simulink model "Appl_MassageMode_CtrlModel"  (R2018b)
settings: configuration reference "CodeConfig_10_ms" (kept outside this file)
undefined symbols (not defined in the file): D_ActMax, D_T1, D_T2, D_T3, D_T4, enMassageLevel_DSM, FALSE, TRUE
libraries: DareLib x33, simulink x1
settings Model: Creator=Administrator  LastModifiedBy=Administrator
settings ConfigSetRef: SourceLocation=Base Workspace

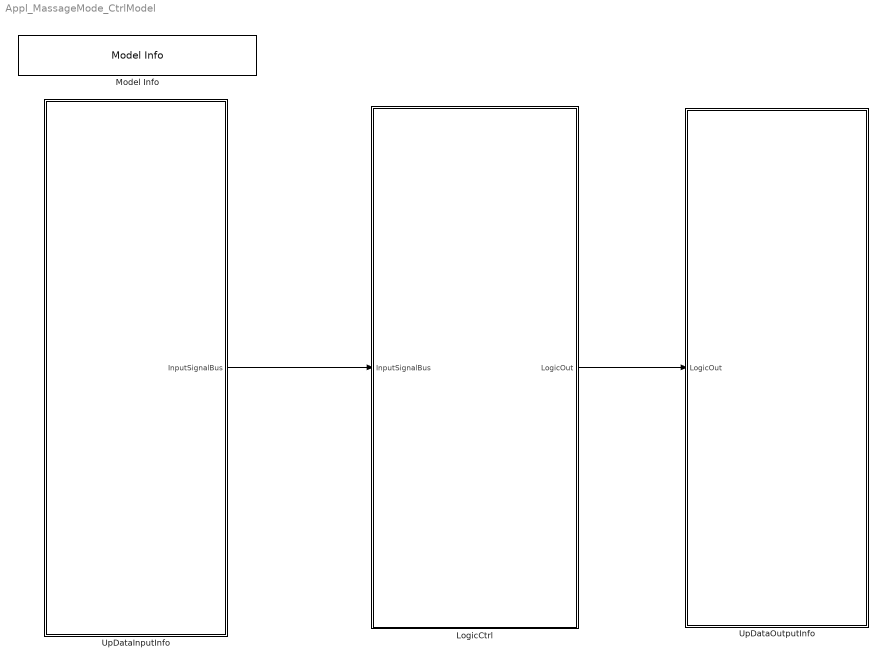
== system Appl_MassageMode_CtrlModel ==
  LogicCtrl : Subsystem  Priority=2  TreatAsAtomicUnit=on
      settings: RTWSystemCode=Nonreusable function  RTWFcnNameOpts=Use subsystem name
  Model Info : simulink/Model-Wide Utilities/Model Info  Frame=on  DisplayStringWithTags=Version：%<ModelVersion>  HorizontalTextAlignment=Center  LeftAlignmentValue=0.5
  UpDataInputInfo : Subsystem  Priority=1  TreatAsAtomicUnit=on
      settings: RTWSystemCode=Nonreusable function  RTWFcnNameOpts=Use subsystem name
  UpDataOutputInfo : Subsystem  Priority=3  TreatAsAtomicUnit=on
      settings: RTWSystemCode=Nonreusable function  RTWFcnNameOpts=Use subsystem name
  wires:
  LogicCtrl/1(LogicOut) -> UpDataOutputInfo/1(LogicOut)
  UpDataInputInfo/1(InputSignalBus) -> LogicCtrl/1(InputSignalBus)

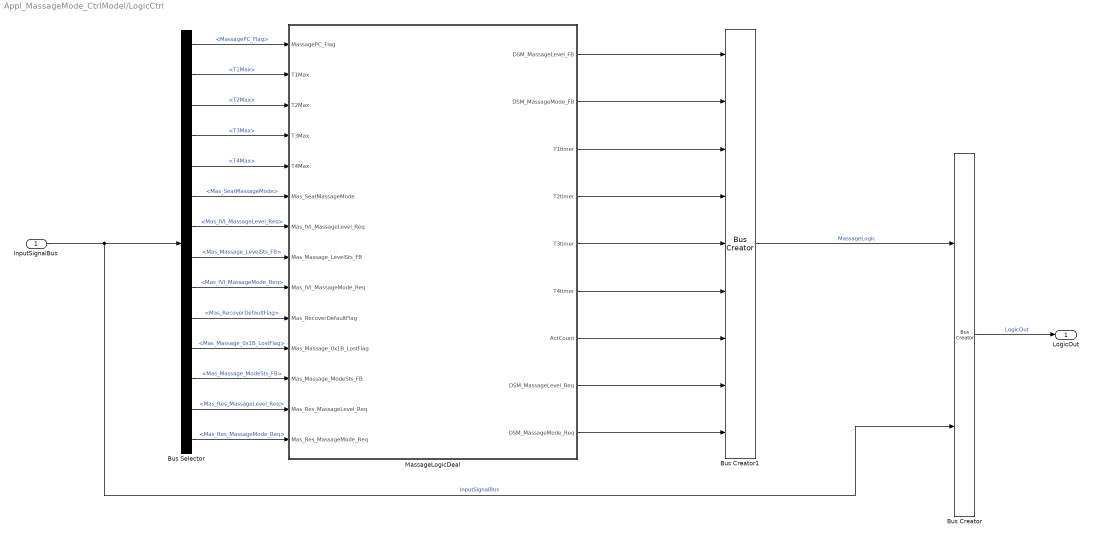
== system Appl_MassageMode_CtrlModel/LogicCtrl ==
  InputSignalBus : Inport
  Bus Creator : BusCreator  Inputs=2
  Bus Creator1 : BusCreator  Inputs=9
  Bus Selector : BusSelector  OutputSignals=MassagePrecondition.MassagePC_Flag,Threshold.T1Max,Threshold.T2Max,Threshold.T3Max,Threshold.T4Max,Rte_SignalBus1.Mas_SeatMassageMode,Rte_SignalBus1.Mas_IVI_MassageLevel_Req,Mas_Massage_LevelSts_FB,Rte_SignalBus1.Mas_IVI_MassageMode_Req,Rte_SignalBus1.Mas_RecoverDefaultFlag,Rte_SignalBus1.Mas_Massage_0x1B_LostFlag,Rte_SignalBus1.Mas_Massage_ModeSts_FB,Rte_SignalBus1.Mas_Res_MassageLevel_Req,Rte_SignalBus1.Mas_Res_MassageMode_Req
  MassageLogicDeal : Subsystem  Description=按摩逻辑处理
      settings: AttributesFormatString=%<Description>
  LogicOut : Outport
  wires:
  InputSignalBus/1 -> Bus Creator/2, Bus Selector/1  "InputSignalBus"
  Bus Creator/1 -> LogicOut/1  "LogicOut"
  MassageLogicDeal/7(ActCount) -> Bus Creator1/7
  MassageLogicDeal/6(T4timer) -> Bus Creator1/6
  MassageLogicDeal/8(DSM_MassageLevel_Req) -> Bus Creator1/8
  MassageLogicDeal/5(T3timer) -> Bus Creator1/5
  MassageLogicDeal/9(DSM_MassageMode_Req) -> Bus Creator1/9
  MassageLogicDeal/4(T2timer) -> Bus Creator1/4
  MassageLogicDeal/3(T1timer) -> Bus Creator1/3
  MassageLogicDeal/2(DSM_MassageMode_FB) -> Bus Creator1/2
  MassageLogicDeal/1(DSM_MassageLevel_FB) -> Bus Creator1/1
  Bus Creator1/1 -> Bus Creator/1  "MassageLogic"
  Bus Selector/1 -> MassageLogicDeal/1(MassagePC_Flag)  "<MassagePC_Flag>"
  Bus Selector/2 -> MassageLogicDeal/2(T1Max)  "<T1Max>"
  Bus Selector/3 -> MassageLogicDeal/3(T2Max)  "<T2Max>"
  Bus Selector/4 -> MassageLogicDeal/4(T3Max)  "<T3Max>"
  Bus Selector/5 -> MassageLogicDeal/5(T4Max)  "<T4Max>"
  Bus Selector/6 -> MassageLogicDeal/6(Mas_SeatMassageMode)  "<Mas_SeatMassageMode>"
  Bus Selector/7 -> MassageLogicDeal/7(Mas_IVI_MassageLevel_Req)  "<Mas_IVI_MassageLevel_Req>"
  Bus Selector/8 -> MassageLogicDeal/8(Mas_Massage_LevelSts_FB)  "<Mas_Massage_LevelSts_FB>"
  Bus Selector/9 -> MassageLogicDeal/9(Mas_IVI_MassageMode_Req)  "<Mas_IVI_MassageMode_Req>"
  Bus Selector/10 -> MassageLogicDeal/10(Mas_RecoverDefaultFlag)  "<Mas_RecoverDefaultFlag>"
  Bus Selector/11 -> MassageLogicDeal/11(Mas_Massage_0x1B_LostFlag)  "<Mas_Massage_0x1B_LostFlag>"
  Bus Selector/12 -> MassageLogicDeal/12(Mas_Massage_ModeSts_FB)  "<Mas_Massage_ModeSts_FB>"
  Bus Selector/13 -> MassageLogicDeal/13(Mas_Res_MassageLevel_Req)  "<Mas_Res_MassageLevel_Req>"
  Bus Selector/14 -> MassageLogicDeal/14(Mas_Res_MassageMode_Req)  "<Mas_Res_MassageMode_Req>"

== system Appl_MassageMode_CtrlModel/UpDataInputInfo ==
  InputSignalProcess : Subsystem  Description=预处理
      settings: AttributesFormatString=%<Description>  RTWSystemCode=Nonreusable function  RTWFcnNameOpts=Use subsystem name
  RTE : Subsystem  Description=接口自动生成  TreatAsAtomicUnit=on
      settings: AttributesFormatString=%<Description>  RTWSystemCode=Nonreusable function  RTWFcnNameOpts=Use subsystem name
  InputSignalBus : Outport
  wires:
  RTE/1(RTE_Signal) -> InputSignalProcess/1(Rte_SignalBus)
  InputSignalProcess/1(InputSignalBus) -> InputSignalBus/1

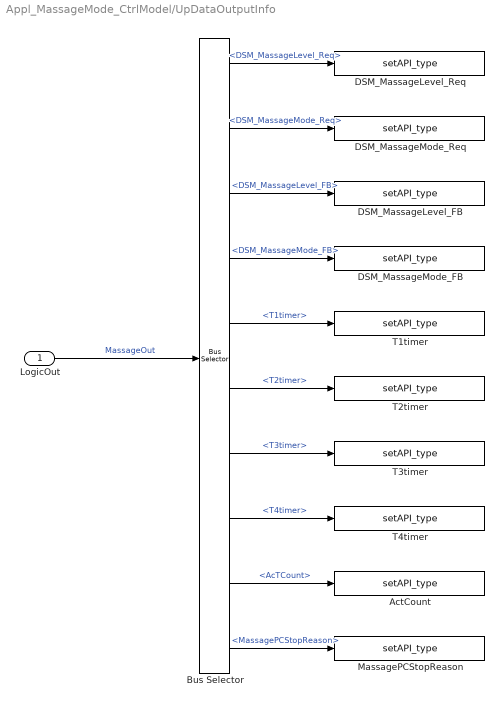
== system Appl_MassageMode_CtrlModel/UpDataOutputInfo ==
  LogicOut : Inport
  ActCount : DareLib/Dare/setAPI_type  g_funcname=Rte_SetVfb_Debug_Mas_ActCount  g_param=""  g_type=uint8  g_size=-1
      settings: AttributesFormatString=%<g_funcname>  SourceProductName=Dare Library
  Bus Selector : BusSelector  OutputSignals=MassageLogic.DSM_MassageLevel_Req,MassageLogic.DSM_MassageMode_Req,MassageLogic.DSM_MassageLevel_FB,MassageLogic.DSM_MassageMode_FB,MassageLogic.T1timer,MassageLogic.T2timer,MassageLogic.T3timer,MassageLogic.T4timer,MassageLogic.AcTCount,InputSignalBus.MassagePrecondition.MassagePCStopReason
  DSM_MassageLevel_FB : DareLib/Dare/setAPI_type  g_funcname=CanTx_0x3B2_DSM_MassageLevel_FB  g_param=""  g_type=uint8  g_enum=enMassageLevel_DSM  g_size=-1
      settings: AttributesFormatString=%<g_funcname>  SourceProductName=Dare Library
  DSM_MassageLevel_Req : DareLib/Dare/setAPI_type  g_funcname=LinSignalSet_DSM_1_1_DSM_MassageLevel_Req  g_param=""  g_type=uint8  g_enum=enMassageLevel_DSM  g_size=-1
      settings: AttributesFormatString=%<g_funcname>  SourceProductName=Dare Library
  DSM_MassageMode_FB : DareLib/Dare/setAPI_type  g_funcname=CanTx_0x3B2_DSM_MassageMode_FB  g_param=""  g_type=uint8  g_enum=enMassageMode_DSM  g_size=-1
      settings: AttributesFormatString=%<g_funcname>  SourceProductName=Dare Library
  DSM_MassageMode_Req : DareLib/Dare/setAPI_type  g_funcname=LinSignalSet_DSM_1_1_DSM_MassageMode_Req  g_param=""  g_type=uint8  g_enum=enMassageMode_DSM  g_size=-1
      settings: AttributesFormatString=%<g_funcname>  SourceProductName=Dare Library
  MassagePCStopReason : DareLib/Dare/setAPI_type  g_funcname=Rte_SetVfb_Debug_Mas_MassagePCStopReason  g_param=""  g_type=uint8  g_size=-1
      settings: AttributesFormatString=%<g_funcname>  SourceProductName=Dare Library
  T1timer : DareLib/Dare/setAPI_type  g_funcname=Rte_SetVfb_Debug_Mas_T1timer  g_param=""  g_type=uint16  g_size=-1
      settings: AttributesFormatString=%<g_funcname>  SourceProductName=Dare Library
  T2timer : DareLib/Dare/setAPI_type  g_funcname=Rte_SetVfb_Debug_Mas_T2timer  g_param=""  g_type=uint16  g_size=-1
      settings: AttributesFormatString=%<g_funcname>  SourceProductName=Dare Library
  T3timer : DareLib/Dare/setAPI_type  g_funcname=Rte_SetVfb_Debug_Mas_T3timer  g_param=""  g_type=uint32  g_size=-1
      settings: AttributesFormatString=%<g_funcname>  SourceProductName=Dare Library
  T4timer : DareLib/Dare/setAPI_type  g_funcname=Rte_SetVfb_Debug_Mas_T4timer  g_param=""  g_type=uint32  g_size=-1
      settings: AttributesFormatString=%<g_funcname>  SourceProductName=Dare Library
  wires:
  LogicOut/1 -> Bus Selector/1  "MassageOut"
  Bus Selector/4 -> DSM_MassageMode_FB/1  "<DSM_MassageMode_FB>"
  Bus Selector/3 -> DSM_MassageLevel_FB/1  "<DSM_MassageLevel_FB>"
  Bus Selector/5 -> T1timer/1  "<T1timer>"
  Bus Selector/2 -> DSM_MassageMode_Req/1  "<DSM_MassageMode_Req>"
  Bus Selector/6 -> T2timer/1  "<T2timer>"
  Bus Selector/1 -> DSM_MassageLevel_Req/1  "<DSM_MassageLevel_Req>"
  Bus Selector/7 -> T3timer/1  "<T3timer>"
  Bus Selector/8 -> T4timer/1  "<T4timer>"
  Bus Selector/9 -> ActCount/1  "<AcTCount>"
  Bus Selector/10 -> MassagePCStopReason/1  "<MassagePCStopReason>"

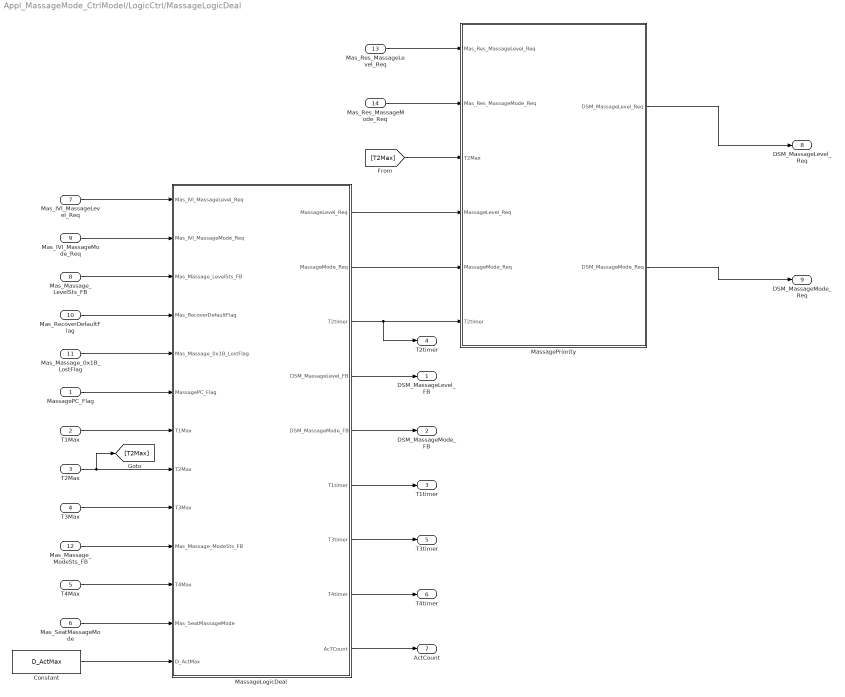
== system Appl_MassageMode_CtrlModel/LogicCtrl/MassageLogicDeal ==
  MassagePC_Flag : Inport
  T1Max : Inport  Port=2
  T2Max : Inport  Port=3
  T3Max : Inport  Port=4
  T4Max : Inport  Port=5
  Mas_SeatMassageMode : Inport  Port=6
  Mas_IVI_MassageLevel_Req : Inport  Port=7
  Mas_Massage_LevelSts_FB : Inport  Port=8
  Mas_IVI_MassageMode_Req : Inport  Port=9
  Mas_RecoverDefaultFlag : Inport  Port=10
  Mas_Massage_0x1B_LostFlag : Inport  Port=11
  Mas_Massage_ModeSts_FB : Inport  Port=12
  Mas_Res_MassageLevel_Req : Inport  Port=13
  Mas_Res_MassageMode_Req : Inport  Port=14
  Constant : Constant  Value=D_ActMax
  MassageLogicDeal : Stateflow chart  TreatAsAtomicUnit=on
  MassagePriority : Stateflow chart  TreatAsAtomicUnit=on
  DSM_MassageLevel_FB : Outport
  DSM_MassageMode_FB : Outport  Port=2
  T1timer : Outport  Port=3
  T2timer : Outport  Port=4
  T3timer : Outport  Port=5
  T4timer : Outport  Port=6
  ActCount : Outport  Port=7
  DSM_MassageLevel_Req : Outport  Port=8
  DSM_MassageMode_Req : Outport  Port=9
  wires:
  MassagePC_Flag/1 -> MassageLogicDeal/6(MassagePC_Flag)
  T1Max/1 -> MassageLogicDeal/7(T1Max)
  T2Max/1 -> [T2Max], MassageLogicDeal/8(T2Max)
  T3Max/1 -> MassageLogicDeal/9(T3Max)
  T4Max/1 -> MassageLogicDeal/11(T4Max)
  MassageLogicDeal/1(MassageLevel_Req) -> MassagePriority/4(MassageLevel_Req)
  MassageLogicDeal/2(MassageMode_Req) -> MassagePriority/5(MassageMode_Req)
  MassageLogicDeal/4(DSM_MassageLevel_FB) -> DSM_MassageLevel_FB/1
  Mas_IVI_MassageMode_Req/1 -> MassageLogicDeal/2(Mas_IVI_MassageMode_Req)
  Mas_RecoverDefaultFlag/1 -> MassageLogicDeal/4(Mas_RecoverDefaultFlag)
  Mas_Massage_0x1B_LostFlag/1 -> MassageLogicDeal/5(Mas_Massage_0x1B_LostFlag)
  Mas_Massage_ModeSts_FB/1 -> MassageLogicDeal/10(Mas_Massage_ModeSts_FB)
  Mas_Massage_LevelSts_FB/1 -> MassageLogicDeal/3(Mas_Massage_LevelSts_FB)
  Mas_IVI_MassageLevel_Req/1 -> MassageLogicDeal/1(Mas_IVI_MassageLevel_Req)
  MassageLogicDeal/7(T3timer) -> T3timer/1
  MassageLogicDeal/3(T2timer) -> T2timer/1, MassagePriority/6(T2timer)
  MassageLogicDeal/6(T1timer) -> T1timer/1
  MassageLogicDeal/5(DSM_MassageMode_FB) -> DSM_MassageMode_FB/1
  Mas_SeatMassageMode/1 -> MassageLogicDeal/12(Mas_SeatMassageMode)
  MassageLogicDeal/8(T4timer) -> T4timer/1
  MassageLogicDeal/9(AcTCount) -> ActCount/1
  Constant/1 -> MassageLogicDeal/13(D_ActMax)
  MassagePriority/2(DSM_MassageMode_Req) -> DSM_MassageMode_Req/1
  MassagePriority/1(DSM_MassageLevel_Req) -> DSM_MassageLevel_Req/1
  Mas_Res_MassageLevel_Req/1 -> MassagePriority/1(Mas_Res_MassageLevel_Req)
  Mas_Res_MassageMode_Req/1 -> MassagePriority/2(Mas_Res_MassageMode_Req)
  [T2Max] -> MassagePriority/3(T2Max)

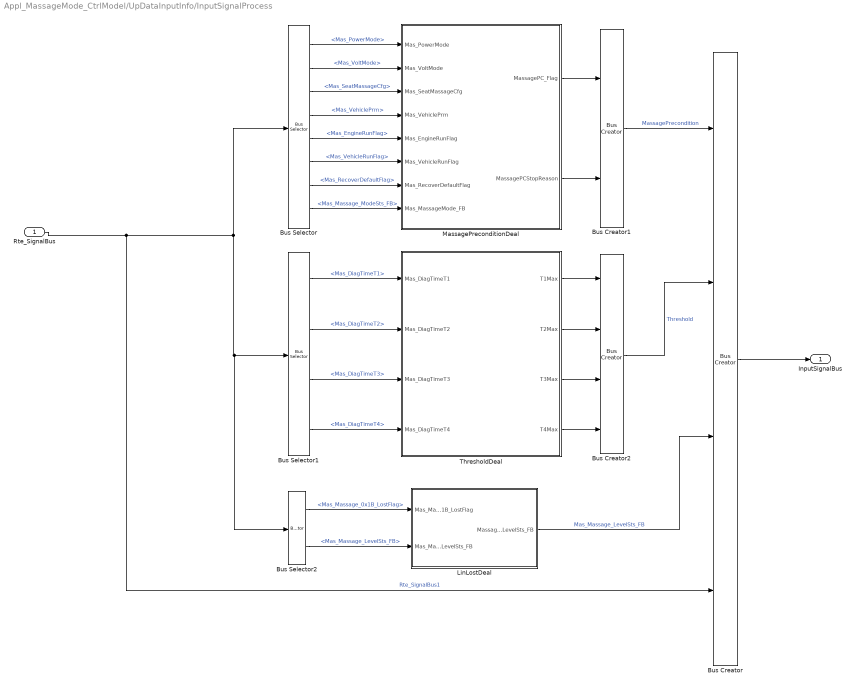
== system Appl_MassageMode_CtrlModel/UpDataInputInfo/InputSignalProcess ==
  Rte_SignalBus : Inport
  Bus Creator : BusCreator  Inputs=4
  Bus Creator1 : BusCreator  Inputs=2
  Bus Creator2 : BusCreator  Inputs=4
  Bus Selector : BusSelector  OutputSignals=Mas_PowerMode,Mas_VoltMode,Mas_SeatMassageCfg,Mas_VehiclePrm,Mas_EngineRunFlag,Mas_VehicleRunFlag,Mas_RecoverDefaultFlag,Mas_Massage_ModeSts_FB
  Bus Selector1 : BusSelector  OutputSignals=Mas_DiagTimeT1,Mas_DiagTimeT2,Mas_DiagTimeT3,Mas_DiagTimeT4
  Bus Selector2 : BusSelector  OutputSignals=Mas_Massage_0x1B_LostFlag,Mas_Massage_LevelSts_FB
  LinLostDeal : Subsystem  Description=LIN节点掉线处理
      settings: AttributesFormatString=%<Description>
  MassagePreconditionDeal : Subsystem  Description=按摩前置条件处理
      settings: AttributesFormatString=%<Description>
  ThresholdDeal : Subsystem  Description=时间阈值配置处理
      settings: AttributesFormatString=%<Description>
  InputSignalBus : Outport
  wires:
  Bus Creator/1 -> InputSignalBus/1
  Rte_SignalBus/1 -> Bus Creator/4, Bus Selector/1, Bus Selector2/1, Bus Selector1/1  "Rte_SignalBus1"
  MassagePreconditionDeal/1(MassagePC_Flag) -> Bus Creator1/1
  MassagePreconditionDeal/2(MassagePCStopReason) -> Bus Creator1/2
  Bus Selector1/1 -> ThresholdDeal/1(Mas_DiagTimeT1)  "<Mas_DiagTimeT1>"
  Bus Selector1/2 -> ThresholdDeal/2(Mas_DiagTimeT2)  "<Mas_DiagTimeT2>"
  Bus Selector1/3 -> ThresholdDeal/3(Mas_DiagTimeT3)  "<Mas_DiagTimeT3>"
  Bus Selector1/4 -> ThresholdDeal/4(Mas_DiagTimeT4)  "<Mas_DiagTimeT4>"
  ThresholdDeal/1(T1Max) -> Bus Creator2/1
  ThresholdDeal/2(T2Max) -> Bus Creator2/2
  ThresholdDeal/3(T3Max) -> Bus Creator2/3
  ThresholdDeal/4(T4Max) -> Bus Creator2/4
  Bus Selector/1 -> MassagePreconditionDeal/1(Mas_PowerMode)  "<Mas_PowerMode>"
  Bus Selector/2 -> MassagePreconditionDeal/2(Mas_VoltMode)  "<Mas_VoltMode>"
  Bus Selector/3 -> MassagePreconditionDeal/3(Mas_SeatMassageCfg)  "<Mas_SeatMassageCfg>"
  Bus Selector/4 -> MassagePreconditionDeal/4(Mas_VehiclePrm)  "<Mas_VehiclePrm>"
  Bus Selector/5 -> MassagePreconditionDeal/5(Mas_EngineRunFlag)  "<Mas_EngineRunFlag>"
  Bus Selector/6 -> MassagePreconditionDeal/6(Mas_VehicleRunFlag)  "<Mas_VehicleRunFlag>"
  Bus Selector/7 -> MassagePreconditionDeal/7(Mas_RecoverDefaultFlag)  "<Mas_RecoverDefaultFlag>"
  Bus Selector/8 -> MassagePreconditionDeal/8(Mas_MassageMode_FB)  "<Mas_Massage_ModeSts_FB>"
  Bus Creator1/1 -> Bus Creator/1  "MassagePrecondition"
  Bus Creator2/1 -> Bus Creator/2  "Threshold"
  Bus Selector2/1 -> LinLostDeal/1(Mas_Massage_0x1B_LostFlag)  "<Mas_Massage_0x1B_LostFlag>"
  Bus Selector2/2 -> LinLostDeal/2(Mas_Massage_LevelSts_FB)  "<Mas_Massage_LevelSts_FB>"
  LinLostDeal/1(Massage_LevelSts_FB) -> Bus Creator/3  "Mas_Massage_LevelSts_FB"

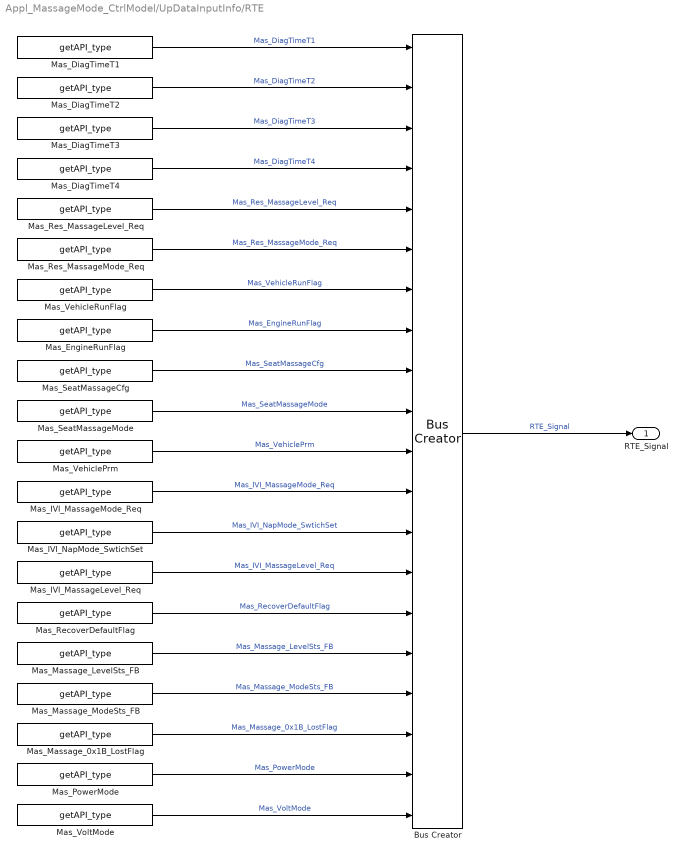
== system Appl_MassageMode_CtrlModel/UpDataInputInfo/RTE ==
  Bus Creator : BusCreator  Inputs=20
  Mas_DiagTimeT1 : DareLib/Dare/getAPI_type  g_funcname=Rte_GetVfb_Debug_Mas_T1_Threshold  g_param=""  g_type=uint16  g_size=-1
      settings: AttributesFormatString=%<g_funcname>  SourceProductName=Dare Library
  Mas_DiagTimeT2 : DareLib/Dare/getAPI_type  g_funcname=Rte_GetVfb_Debug_Mas_T2_Threshold  g_param=""  g_type=uint16  g_size=-1
      settings: AttributesFormatString=%<g_funcname>  SourceProductName=Dare Library
  Mas_DiagTimeT3 : DareLib/Dare/getAPI_type  g_funcname=Rte_GetVfb_Debug_Mas_T3_Threshold  g_param=""  g_type=uint16  g_size=-1
      settings: AttributesFormatString=%<g_funcname>  SourceProductName=Dare Library
  Mas_DiagTimeT4 : DareLib/Dare/getAPI_type  g_funcname=Rte_GetVfb_Debug_Mas_T4_Threshold  g_param=""  g_type=uint16  g_size=-1
      settings: AttributesFormatString=%<g_funcname>  SourceProductName=Dare Library
  Mas_EngineRunFlag : DareLib/Dare/getAPI_type  g_funcname=Rte_GetVfb_EngineRunFlag  g_param=""  g_type=uint8  g_size=-1
      settings: AttributesFormatString=%<g_funcname>  SourceProductName=Dare Library
  Mas_IVI_MassageLevel_Req : DareLib/Dare/getAPI_type  g_funcname=CanRx_0x351_IVI_MassageLevel_Req  g_param=""  g_type=uint8  g_enum=enMassageLevel_IVI  g_size=-1
      settings: AttributesFormatString=%<g_funcname>  SourceProductName=Dare Library
  Mas_IVI_MassageMode_Req : DareLib/Dare/getAPI_type  g_funcname=CanRx_0x351_IVI_MassageMode_Req  g_param=""  g_type=uint8  g_enum=enMassageMode_IVI  g_size=-1
      settings: AttributesFormatString=%<g_funcname>  SourceProductName=Dare Library
  Mas_IVI_NapMode_SwtichSet : DareLib/Dare/getAPI_type  g_funcname=CanRx_0x367_IVI_NapMode_SwtichSet  g_param=""  g_type=uint8  g_size=-1
      settings: AttributesFormatString=%<g_funcname>  SourceProductName=Dare Library
  Mas_Massage_0x1B_LostFlag : DareLib/Dare/getAPI_type  g_funcname=Ecual_LinGetLostPid  g_param=""  g_type=uint8  g_size=-1
      settings: AttributesFormatString=%<g_funcname>  SourceProductName=Dare Library
  Mas_Massage_LevelSts_FB : DareLib/Dare/getAPI_type  g_funcname=LinSignalGet_Massage_1_Massage_LevelSts_FB  g_param=""  g_type=uint8  g_enum=enMassageLevel_DSM  g_size=-1
      settings: AttributesFormatString=%<g_funcname>  SourceProductName=Dare Library
  Mas_Massage_ModeSts_FB : DareLib/Dare/getAPI_type  g_funcname=LinSignalGet_Massage_1_Massage_ModeSts_FB  g_param=""  g_type=uint8  g_enum=enMassageMode_DSM  g_size=-1
      settings: AttributesFormatString=%<g_funcname>  SourceProductName=Dare Library
  Mas_PowerMode : DareLib/Dare/getAPI_type  g_funcname=Rte_GetVfb_PowerMode  g_param=""  g_type=uint8  g_enum=enPowerModeSts  g_size=-1
      settings: AttributesFormatString=%<g_funcname>  SourceProductName=Dare Library
  Mas_RecoverDefaultFlag : DareLib/Dare/getAPI_type  g_funcname=GetRecoverDefaultFlag  g_param=""  g_type=uint8  g_size=-1
      settings: AttributesFormatString=%<g_funcname>  SourceProductName=Dare Library
  Mas_Res_MassageLevel_Req : DareLib/Dare/getAPI_type  g_funcname=Rte_GetVfb_Res_MassageLevel_Req  g_param=""  g_type=uint8  g_enum=enMassageLevel_DSM  g_size=-1
      settings: AttributesFormatString=%<g_funcname>  SourceProductName=Dare Library
  Mas_Res_MassageMode_Req : DareLib/Dare/getAPI_type  g_funcname=Rte_GetVfb_Res_MassageMode_Req  g_param=""  g_type=uint8  g_enum=enMassageMode_DSM  g_size=-1
      settings: AttributesFormatString=%<g_funcname>  SourceProductName=Dare Library
  Mas_SeatMassageCfg : DareLib/Dare/getAPI_type  g_funcname=Srvl_GetMemIndexDataU8  g_param=EN_MemIndex_MassageConfig  g_type=uint8  g_size=-1
      settings: AttributesFormatString=%<g_funcname>  SourceProductName=Dare Library
  Mas_SeatMassageMode : DareLib/Dare/getAPI_type  g_funcname=Srvl_GetMemIndexDataU8  g_param=EN_MemIndex_MassageMode  g_type=uint8  g_enum=enMassageMode_DSM  g_size=-1
      settings: AttributesFormatString=%<g_funcname>  SourceProductName=Dare Library
  Mas_VehiclePrm : DareLib/Dare/getAPI_type  g_funcname=Srvl_GetMemIndexDataU8  g_param=EN_MemIndex_Heat_CarType  g_type=uint8  g_enum=enVehTypePrm  g_size=-1
      settings: AttributesFormatString=%<g_funcname>  SourceProductName=Dare Library
  Mas_VehicleRunFlag : DareLib/Dare/getAPI_type  g_funcname=Rte_GetVfb_VehicleRunFlag  g_param=""  g_type=uint8  g_size=-1
      settings: AttributesFormatString=%<g_funcname>  SourceProductName=Dare Library
  Mas_VoltMode : DareLib/Dare/getAPI_type  g_funcname=Rte_GetVfb_VoltMode  g_param=""  g_type=uint8  g_enum=enFinalPowerMode  g_size=-1
      settings: AttributesFormatString=%<g_funcname>  SourceProductName=Dare Library
  RTE_Signal : Outport
  wires:
  Bus Creator/1 -> RTE_Signal/1  "RTE_Signal"
  Mas_DiagTimeT1/1 -> Bus Creator/1  "Mas_DiagTimeT1"
  Mas_DiagTimeT2/1 -> Bus Creator/2  "Mas_DiagTimeT2"
  Mas_DiagTimeT3/1 -> Bus Creator/3  "Mas_DiagTimeT3"
  Mas_DiagTimeT4/1 -> Bus Creator/4  "Mas_DiagTimeT4"
  Mas_Res_MassageLevel_Req/1 -> Bus Creator/5  "Mas_Res_MassageLevel_Req"
  Mas_Res_MassageMode_Req/1 -> Bus Creator/6  "Mas_Res_MassageMode_Req"
  Mas_VehicleRunFlag/1 -> Bus Creator/7  "Mas_VehicleRunFlag"
  Mas_EngineRunFlag/1 -> Bus Creator/8  "Mas_EngineRunFlag"
  Mas_SeatMassageCfg/1 -> Bus Creator/9  "Mas_SeatMassageCfg"
  Mas_SeatMassageMode/1 -> Bus Creator/10  "Mas_SeatMassageMode"
  Mas_VehiclePrm/1 -> Bus Creator/11  "Mas_VehiclePrm"
  Mas_IVI_MassageMode_Req/1 -> Bus Creator/12  "Mas_IVI_MassageMode_Req"
  Mas_IVI_NapMode_SwtichSet/1 -> Bus Creator/13  "Mas_IVI_NapMode_SwtichSet"
  Mas_IVI_MassageLevel_Req/1 -> Bus Creator/14  "Mas_IVI_MassageLevel_Req"
  Mas_RecoverDefaultFlag/1 -> Bus Creator/15  "Mas_RecoverDefaultFlag"
  Mas_Massage_LevelSts_FB/1 -> Bus Creator/16  "Mas_Massage_LevelSts_FB"
  Mas_Massage_ModeSts_FB/1 -> Bus Creator/17  "Mas_Massage_ModeSts_FB"
  Mas_Massage_0x1B_LostFlag/1 -> Bus Creator/18  "Mas_Massage_0x1B_LostFlag"
  Mas_PowerMode/1 -> Bus Creator/19  "Mas_PowerMode"
  Mas_VoltMode/1 -> Bus Creator/20  "Mas_VoltMode"

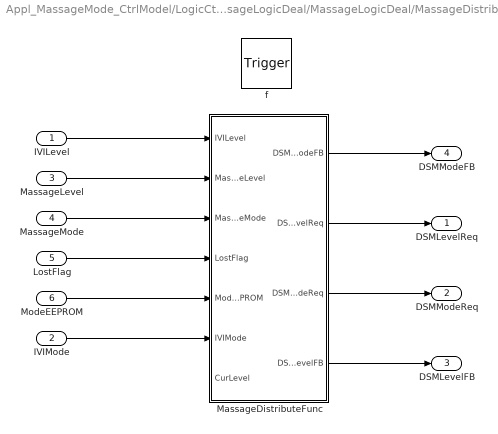
== system Appl_MassageMode_CtrlModel/LogicCtrl/MassageLogicDeal/MassageLogicDeal/MassageDistributeFunc ==
  IVILevel : Inport
  IVIMode : Inport  Port=2
  MassageLevel : Inport  Port=3
  MassageMode : Inport  Port=4
  LostFlag : Inport  Port=5
  ModeEEPROM : Inport  Port=6
  f : TriggerPort  TriggerType=function-call  VariantControl=(inherit)
      settings: CopyFcn=Stateflow.SLINSF.SimulinkMan.removeBlockPreDeleteFcn  PreDeleteFcn=Stateflow.SLINSF.SimulinkMan.unsafePredeleteFcn
  MassageDistributeFunc : Stateflow chart  TreatAsAtomicUnit=on
  DSMLevelReq : Outport
  DSMModeReq : Outport  Port=2
  DSMLevelFB : Outport  Port=3
  DSMModeFB : Outport  Port=4
  wires:
  IVILevel/1 -> MassageDistributeFunc/1(IVILevel)
  IVIMode/1 -> MassageDistributeFunc/6(IVIMode)
  MassageLevel/1 -> MassageDistributeFunc/2(MassageLevel)
  MassageMode/1 -> MassageDistributeFunc/3(MassageMode)
  LostFlag/1 -> MassageDistributeFunc/4(LostFlag)
  ModeEEPROM/1 -> MassageDistributeFunc/5(ModeEEPROM)
  MassageDistributeFunc/1(DSMModeFB) -> DSMModeFB/1
  MassageDistributeFunc/2(DSMLevelReq) -> DSMLevelReq/1
  MassageDistributeFunc/3(DSMModeReq) -> DSMModeReq/1
  MassageDistributeFunc/4(DSMLevelFB) -> DSMLevelFB/1
  ? -> MassageDistributeFunc/7(CurLevel)

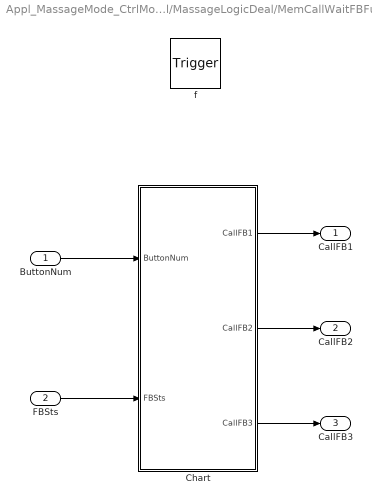
== system Appl_MassageMode_CtrlModel/LogicCtrl/MassageLogicDeal/MassageLogicDeal/MemCallWaitFBFunc ==
  ButtonNum : Inport
  FBSts : Inport  Port=2
  f : TriggerPort  TriggerType=function-call  VariantControl=(inherit)
      settings: CopyFcn=Stateflow.SLINSF.SimulinkMan.removeBlockPreDeleteFcn  PreDeleteFcn=Stateflow.SLINSF.SimulinkMan.unsafePredeleteFcn
  Chart : Stateflow chart  TreatAsAtomicUnit=on
  CallFB1 : Outport
  CallFB2 : Outport  Port=2
  CallFB3 : Outport  Port=3
  wires:
  ButtonNum/1 -> Chart/1(ButtonNum)
  FBSts/1 -> Chart/2(FBSts)
  Chart/1(CallFB1) -> CallFB1/1
  Chart/2(CallFB2) -> CallFB2/1
  Chart/3(CallFB3) -> CallFB3/1

== system Appl_MassageMode_CtrlModel/LogicCtrl/MassageLogicDeal/MassagePriority/SaveMassageMode ==
  Mode : Inport
  f : TriggerPort  TriggerType=function-call  VariantControl=(inherit)
      settings: CopyFcn=Stateflow.SLINSF.SimulinkMan.removeBlockPreDeleteFcn  PreDeleteFcn=Stateflow.SLINSF.SimulinkMan.unsafePredeleteFcn
  setAPI_type3 : DareLib/Dare/setAPI_type  g_funcname=Srvl_SetMemIndexDataU8  g_param=EN_MemIndex_MassageMode  g_type=uint8  g_enum=enMassageMode_DSM  g_size=-1
      settings: AttributesFormatString=%<g_funcname>  SourceProductName=Dare Library
  wires:
  Mode/1 -> setAPI_type3/1

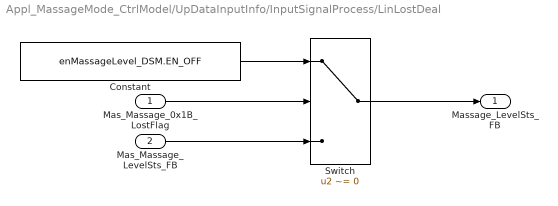
== system Appl_MassageMode_CtrlModel/UpDataInputInfo/InputSignalProcess/LinLostDeal ==
  Mas_Massage_0x1B_LostFlag : Inport
  Mas_Massage_LevelSts_FB : Inport  Port=2
  Constant : Constant  Value=enMassageLevel_DSM.EN_OFF
  Switch : Switch  Criteria=u2 ~= 0
  Massage_LevelSts_FB : Outport
  wires:
  Mas_Massage_LevelSts_FB/1 -> Switch/3
  Mas_Massage_0x1B_LostFlag/1 -> Switch/2
  Switch/1 -> Massage_LevelSts_FB/1
  Constant/1 -> Switch/1

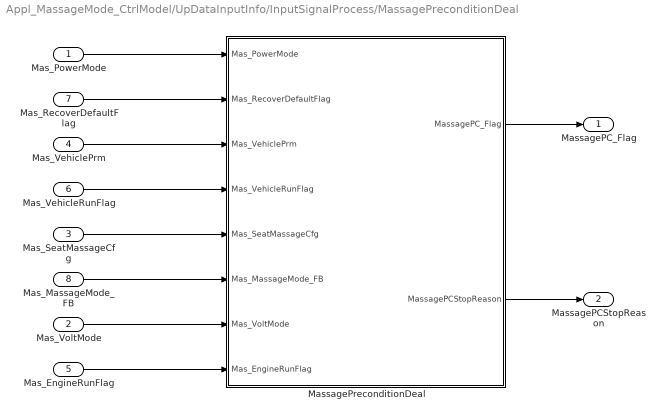
== system Appl_MassageMode_CtrlModel/UpDataInputInfo/InputSignalProcess/MassagePreconditionDeal ==
  Mas_PowerMode : Inport
  Mas_VoltMode : Inport  Port=2
  Mas_SeatMassageCfg : Inport  Port=3
  Mas_VehiclePrm : Inport  Port=4
  Mas_EngineRunFlag : Inport  Port=5
  Mas_VehicleRunFlag : Inport  Port=6
  Mas_RecoverDefaultFlag : Inport  Port=7
  Mas_MassageMode_FB : Inport  Port=8
  MassagePreconditionDeal : Stateflow chart  TreatAsAtomicUnit=on
  MassagePC_Flag : Outport
  MassagePCStopReason : Outport  Port=2
  wires:
  MassagePreconditionDeal/1(MassagePC_Flag) -> MassagePC_Flag/1
  Mas_VehicleRunFlag/1 -> MassagePreconditionDeal/4(Mas_VehicleRunFlag)
  Mas_SeatMassageCfg/1 -> MassagePreconditionDeal/5(Mas_SeatMassageCfg)
  Mas_PowerMode/1 -> MassagePreconditionDeal/1(Mas_PowerMode)
  Mas_RecoverDefaultFlag/1 -> MassagePreconditionDeal/2(Mas_RecoverDefaultFlag)
  Mas_VehiclePrm/1 -> MassagePreconditionDeal/3(Mas_VehiclePrm)
  Mas_EngineRunFlag/1 -> MassagePreconditionDeal/8(Mas_EngineRunFlag)
  Mas_VoltMode/1 -> MassagePreconditionDeal/7(Mas_VoltMode)
  Mas_MassageMode_FB/1 -> MassagePreconditionDeal/6(Mas_MassageMode_FB)
  MassagePreconditionDeal/2(MassagePCStopReason) -> MassagePCStopReason/1

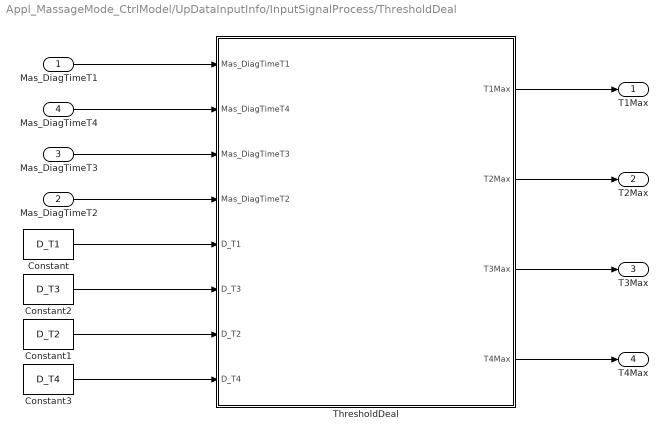
== system Appl_MassageMode_CtrlModel/UpDataInputInfo/InputSignalProcess/ThresholdDeal ==
  Mas_DiagTimeT1 : Inport
  Mas_DiagTimeT2 : Inport  Port=2
  Mas_DiagTimeT3 : Inport  Port=3
  Mas_DiagTimeT4 : Inport  Port=4
  Constant : Constant  Value=D_T1
  Constant1 : Constant  Value=D_T2
  Constant2 : Constant  Value=D_T3
  Constant3 : Constant  Value=D_T4
  ThresholdDeal : Stateflow chart  TreatAsAtomicUnit=on
  T1Max : Outport
  T2Max : Outport  Port=2
  T3Max : Outport  Port=3
  T4Max : Outport  Port=4
  wires:
  ThresholdDeal/4(T4Max) -> T4Max/1
  ThresholdDeal/3(T3Max) -> T3Max/1
  ThresholdDeal/2(T2Max) -> T2Max/1
  ThresholdDeal/1(T1Max) -> T1Max/1
  Mas_DiagTimeT2/1 -> ThresholdDeal/4(Mas_DiagTimeT2)
  Mas_DiagTimeT3/1 -> ThresholdDeal/3(Mas_DiagTimeT3)
  Mas_DiagTimeT1/1 -> ThresholdDeal/1(Mas_DiagTimeT1)
  Mas_DiagTimeT4/1 -> ThresholdDeal/2(Mas_DiagTimeT4)
  Constant/1 -> ThresholdDeal/5(D_T1)
  Constant1/1 -> ThresholdDeal/7(D_T2)
  Constant2/1 -> ThresholdDeal/6(D_T3)
  Constant3/1 -> ThresholdDeal/8(D_T4)

== system Appl_MassageMode_CtrlModel/LogicCtrl/MassageLogicDeal/MassageLogicDeal/MassageDistributeFunc/MassageDistributeFunc/SaveMassageMode ==
  Mode : Inport
  f : TriggerPort  TriggerType=function-call  VariantControl=(inherit)
      settings: CopyFcn=Stateflow.SLINSF.SimulinkMan.removeBlockPreDeleteFcn  PreDeleteFcn=Stateflow.SLINSF.SimulinkMan.unsafePredeleteFcn
  setAPI_type3 : DareLib/Dare/setAPI_type  g_funcname=Srvl_SetMemIndexDataU8  g_param=EN_MemIndex_MassageMode  g_type=uint8  g_enum=enMassageMode_DSM  g_size=-1
      settings: AttributesFormatString=%<g_funcname>  SourceProductName=Dare Library
  wires:
  Mode/1 -> setAPI_type3/1

== system Appl_MassageMode_CtrlModel/UpDataInputInfo/InputSignalProcess/MassagePreconditionDeal/MassagePreconditionDeal/SaveMassageMode ==
  Mode : Inport
  f : TriggerPort  TriggerType=function-call  VariantControl=(inherit)
      settings: CopyFcn=Stateflow.SLINSF.SimulinkMan.removeBlockPreDeleteFcn  PreDeleteFcn=Stateflow.SLINSF.SimulinkMan.unsafePredeleteFcn
  setAPI_type3 : DareLib/Dare/setAPI_type  g_funcname=Srvl_SetMemIndexDataU8  g_param=EN_MemIndex_MassageMode  g_type=uint8  g_enum=enMassageMode_DSM  g_size=-1
      settings: AttributesFormatString=%<g_funcname>  SourceProductName=Dare Library
  wires:
  Mode/1 -> setAPI_type3/1

== system Appl_MassageMode_CtrlModel/UpDataInputInfo/InputSignalProcess/ThresholdDeal/ThresholdDeal/MassageTimeCaliFunc ==
  DiagTime : Inport
  OrgTime : Inport  Port=2
  f : TriggerPort  TriggerType=function-call  VariantControl=(inherit)
      settings: CopyFcn=Stateflow.SLINSF.SimulinkMan.removeBlockPreDeleteFcn  PreDeleteFcn=Stateflow.SLINSF.SimulinkMan.unsafePredeleteFcn
  MassageTimeCaliFunc : Stateflow chart  TreatAsAtomicUnit=on
  Tmax : Outport
  wires:
  DiagTime/1 -> MassageTimeCaliFunc/1(DiagTime)
  OrgTime/1 -> MassageTimeCaliFunc/2(OrgTime)
  MassageTimeCaliFunc/1(TMax) -> Tmax/1

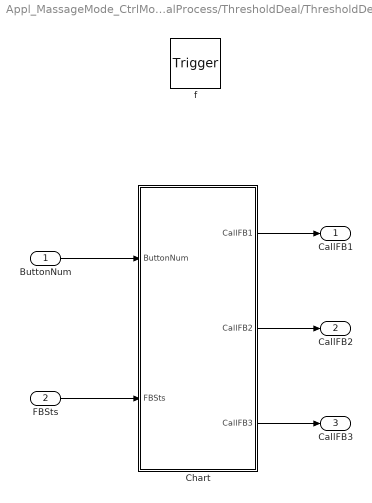
== system Appl_MassageMode_CtrlModel/UpDataInputInfo/InputSignalProcess/ThresholdDeal/ThresholdDeal/MemCallWaitFBFunc ==
  ButtonNum : Inport
  FBSts : Inport  Port=2
  f : TriggerPort  TriggerType=function-call  VariantControl=(inherit)
      settings: CopyFcn=Stateflow.SLINSF.SimulinkMan.removeBlockPreDeleteFcn  PreDeleteFcn=Stateflow.SLINSF.SimulinkMan.unsafePredeleteFcn
  Chart : Stateflow chart  TreatAsAtomicUnit=on
  CallFB1 : Outport
  CallFB2 : Outport  Port=2
  CallFB3 : Outport  Port=3
  wires:
  ButtonNum/1 -> Chart/1(ButtonNum)
  FBSts/1 -> Chart/2(FBSts)
  Chart/1(CallFB1) -> CallFB1/1
  Chart/2(CallFB2) -> CallFB2/1
  Chart/3(CallFB3) -> CallFB3/1

== stateflow chart Appl_MassageMode_CtrlModel/UpDataInputInfo/InputSignalProcess/ThresholdDeal/ThresholdDeal ==
  state [CallFB1,CallFB2,CallFB3] = MemCallWaitFBFunc(ButtonNum,FBSts) [function] [commented out]
  state Tmax  = MassageTimeCaliFunc(DiagTime,OrgTime) [function]
  state Init
    en,du:
    T1Max = MassageTimeCaliFunc(Mas_DiagTimeT1,D_T1);
    T2Max = MassageTimeCaliFunc(Mas_DiagTimeT2,D_T2);
    T3Max = MassageTimeCaliFunc(Mas_DiagTimeT3,D_T3);
    T4Max = MassageTimeCaliFunc(Mas_DiagTimeT4,D_T4);
  (default) -> Init
  data: ButtonNum function_input double size=1; FBSts function_input double size=1; CallFB1 function_output double size=1; CallFB2 function_output double size=1; CallFB3 function_output double size=1; DiagTime function_input; OrgTime function_input; Tmax function_output; TRUE parameter; FALSE parameter; Mas_DiagTimeT1 input; Mas_DiagTimeT4 input; Mas_DiagTimeT3 input; Mas_DiagTimeT2 input; T1Max output uint32; T2Max output uint32; T3Max output uint32; T4Max output uint32; D_T1 input; D_T3 input; D_T2 input; D_T4 input

== stateflow chart Appl_MassageMode_CtrlModel/UpDataInputInfo/InputSignalProcess/ThresholdDeal/ThresholdDeal/MassageTimeCaliFunc/MassageTimeCaliFunc ==
  (default) -> (junction 5)
  (junction 5) -> (junction 7) [order 1] : /* 是否诊断配置 */
      | [DiagTime == 0]
  (junction 5) -> (junction 20) [order 2] : {TMax = DiagTime*100;}
  (junction 7) -> (junction 9) : {TMax = OrgTime;}
  (junction 9) -> (junction 20)
  (junction 20) -> (junction 27)
  data: DiagTime input uint16; OrgTime input uint32; TMax output uint32

== stateflow chart Appl_MassageMode_CtrlModel/LogicCtrl/MassageLogicDeal/MassageLogicDeal/MemCallWaitFBFunc/Chart ==
  (default) -> (junction 3)
  (junction 3) -> (junction 5) : {CallFB1 = enMemCallFb.EN_MemCallFb_NULL;
      | CallFB2 = enMemCallFb.EN_MemCallFb_NULL;
      | CallFB3 = enMemCallFb.EN_MemCallFb_NULL;}
  (junction 5) -> (junction 7) [order 1] : /* 调用位置1进行中 */
      | [ButtonNum == 1]
  (junction 5) -> (junction 14) [order 2]
  (junction 7) -> (junction 9) : {CallFB1 = FBSts;}
  (junction 14) -> (junction 16) [order 1] : /* 调用位置2 进行中 */
      | [ButtonNum == 2]
  (junction 14) -> (junction 20) [order 2] : {CallFB3 = FBSts;}
  (junction 16) -> (junction 18) : {CallFB2 = FBSts;}
  (junction 18) -> (junction 20)
  (junction 9) -> (junction 18)
  (junction 20) -> (junction 27)
  data: ButtonNum input uint8; FBSts input Enum: enMemCallFb; CallFB1 output Enum: enMemCallFb; CallFB2 output Enum: enMemCallFb; CallFB3 output Enum: enMemCallFb

== stateflow chart Appl_MassageMode_CtrlModel/LogicCtrl/MassageLogicDeal/MassageLogicDeal/MassageDistributeFunc/MassageDistributeFunc ==
  note: /* Note
      | 存储 模式 至EEPROM
      | 输入：1.模式 */
  state SaveMassageMode(Mode) [function]
  state IVIModeDistribute [parallel]
    settings: executionOrder=3
    note: IVI节点模式转发
    (default) -> (junction 92)
    IVIModeDistribute -> (junction 92)
    (junction 92) -> (junction 91) [order 1] : /*是否为IVI有效指令&&按摩档位已打开*/
        | [IVIMode <= enMassageMode_IVI.EN_M8 ...
        | && IVIMode != enMassageMode_IVI.EN_Inactive ...
        | && LevelFB != enMassageLevel_DSM.EN_AUTO_OFF ...
        | && LevelFB != enMassageLevel_DSM.EN_OFF]
    (junction 92) -> (junction 96) [order 2] : {DSMModeReq = ModeEEPROM;}
    (junction 91) -> (junction 88) : {DSMModeReq = IVIMode -1;
        | SaveMassageMode(DSMModeReq)}
    (junction 88) -> (junction 96)
    (junction 96) -> (junction 99)
  state IVILevelDistribute [parallel]
    settings: executionOrder=1
    note: IVI节点档位转发
    (default) -> (junction 38)
    IVILevelDistribute -> (junction 38)
    (junction 38) -> (junction 40) [order 1] : /*是否为IVI关闭指令*/
        | [IVILevel == enMassageLevel_IVI.EN_OFF]
    (junction 38) -> (junction 46) [order 2]
    (junction 40) -> (junction 44) : {DSMLevelReq = enMassageLevel_DSM.EN_OFF}
    (junction 46) -> (junction 48) [order 1] : [IVILevel == enMassageLevel_IVI.EN_L1 ...
        | || IVILevel == enMassageLevel_IVI.EN_L2 ...
        | || IVILevel == enMassageLevel_IVI.EN_L3]
    (junction 46) -> (junction 53) [order 2] : {DSMLevelReq = enMassageLevel_DSM.EN_Inactive}
    (junction 48) -> (junction 50) : {DSMLevelReq = IVILevel}
    (junction 50) -> (junction 53)
    (junction 44) -> (junction 50)
    (junction 53) -> (junction 56)
  state MassageModeDistribute [parallel]
    settings: executionOrder=4
    note: Massage节点模式转发
    (default) -> (junction 111)
    MassageModeDistribute -> (junction 111)
    (junction 111) -> (junction 112) [order 1] : /*Massage节点有效指令&&按摩档位已打开*/
        | [MassageMode <= enMassageMode_DSM.EN_MError ...
        | && LevelFB != enMassageLevel_DSM.EN_AUTO_OFF ...
        | && LevelFB != enMassageLevel_DSM.EN_OFF ...
        | && LostFlag != TRUE]
    (junction 111) -> (junction 113) [order 2] : {DSMModeFB = ModeEEPROM;}
    (junction 112) -> (junction 114) : {DSMModeFB = MassageMode;}
    (junction 114) -> (junction 113)
    (junction 113) -> (junction 116)
  state MassageLevelDistribute [parallel]
    settings: executionOrder=2
    note: Massage节点档位转发
    (default) -> (junction 65)
    MassageLevelDistribute -> (junction 65)
    (junction 65) -> (junction 64) [order 1] : /*是否为Massage节点有效指令*/
        | [MassageLevel <= enMassageLevel_DSM.EN_L3]
    (junction 65) -> (junction 79) [order 2]
    (junction 64) -> (junction 61) : {DSMLevelFB = MassageLevel;
        | LevelFB = MassageLevel;}
    (junction 61) -> (junction 79)
    (junction 79) -> (junction 72)
  data: Mode function_input; IVILevel input Enum: enMassageLevel_IVI; MassageLevel input Enum: enMassageLevel_DSM; MassageMode input Enum: enMassageMode_DSM; LostFlag input uint8; ModeEEPROM input Enum: enMassageMode_DSM; IVIMode input Enum: enMassageMode_DSM; DSMModeFB output Enum: enMassageMode_DSM; DSMLevelReq output Enum: enMassageLevel_DSM; DSMModeReq output Enum: enMassageMode_DSM; DSMLevelFB output Enum: enMassageLevel_DSM; LevelFB local Enum: enMassageLevel_DSM; TRUE parameter; CurLevel input Enum: enMassageMode_DSM

== stateflow chart Appl_MassageMode_CtrlModel/LogicCtrl/MassageLogicDeal/MassagePriority ==
  note: /* Note
      | 存储 模式 至EEPROM
      | 输入：1.模式 */
  state SaveMassageMode(Mode) [function]
  state MassagePriority
    (default) -> (junction 175)
    MassagePriority -> (junction 175)
    (junction 175) -> (junction 177) [order 1] : /*(小憩按摩请求变为Level3或OFF)&&未开启T2计时*/
        | [(hasChangedTo(Mas_Res_MassageLevel_Req,enMassageLevel_DSM.EN_L3) ...
        | || hasChangedTo(Mas_Res_MassageLevel_Req,enMassageLevel_DSM.EN_OFF)) ...
        | && (T2timer >= T2Max || T2timer == 0)]
    (junction 177) -> (junction 210) [order 1] : /*开启小憩的时候才更新档位*/
        | [Mas_Res_MassageLevel_Req == enMassageLevel_DSM.EN_L3]
    (junction 175) -> (junction 184) [order 2]
    (junction 177) -> (junction 214) [order 2]
    (junction 210) -> (junction 212) : {DSM_MassageMode_Req = Mas_Res_MassageMode_Req;
        | SaveMassageMode(DSM_MassageMode_Req)}
    (junction 212) -> (junction 214)
    (junction 214) -> (junction 179) : {DSM_MassageLevel_Req = Mas_Res_MassageLevel_Req;}
    (junction 184) -> (junction 186) [order 1] : /*按摩档位*/
        | [hasChangedTo(MassageLevel_Req,enMassageLevel_DSM.EN_OFF) ...
        | ||hasChangedTo(MassageLevel_Req,enMassageLevel_DSM.EN_L1) ...
        | ||hasChangedTo(MassageLevel_Req,enMassageLevel_DSM.EN_L2) ...
        | ||hasChangedTo(MassageLevel_Req,enMassageLevel_DSM.EN_L3) ...
        | ||hasChangedTo(MassageLevel_Req,enMassageLevel_DSM.EN_AUTO_OFF)
        | ]
    (junction 184) -> (junction 191) [order 2]
    (junction 186) -> (junction 188) : {DSM_MassageLevel_Req = MassageLevel_Req;}
    (junction 188) -> (junction 191)
    (junction 191) -> (junction 194)
    (junction 194) -> (junction 198) [order 1] : /*模式请求变化*/
        | [hasChanged(MassageMode_Req)]
    (junction 194) -> (junction 200) [order 2]
    (junction 198) -> (junction 201) : {DSM_MassageMode_Req = MassageMode_Req;}
    (junction 201) -> (junction 200)
    (junction 200) -> (junction 205)
    (junction 179) -> (junction 205)
    (junction 205) -> (junction 208)
  data: Mode function_input; DSM_MassageLevel_Req output Enum: enMassageLevel_DSM; DSM_MassageMode_Req output Enum: enMassageMode_DSM; FALSE parameter; Mas_Res_MassageLevel_Req input; Mas_Res_MassageMode_Req input; T2Max input; MassageLevel_Req input; MassageMode_Req input; TRUE parameter; ResReCallPosi_Back local uint16; ResReCallPosi_Front local uint16; ResReCallPosi_Height local uint16; ResReCallPosi_Length local uint16; T2timer input

== stateflow chart Appl_MassageMode_CtrlModel/LogicCtrl/MassageLogicDeal/MassageLogicDeal ==
  state [CallFB1,CallFB2,CallFB3] = MemCallWaitFBFunc(ButtonNum,FBSts) [function] [commented out]
  note: /* Note
      | 函数说明：按摩档位、模式转发策略
      | 输入：1.IVI档位请求CAN报文；2.IVI模式请求CAN报文；3.Massage档位反馈LIN报文；4.Massage模式反馈LIN报文;5.LIN掉线标志;6.EEPROM中存储的按摩模式;
      | 输出：1.DSM外发档位LIN报文；2.DSM外发模式LIN报文；3.DSM外发档位CAN报文；4.DSM外发模式CAN报文 */
  state [DSMLevelReq,DSMModeReq,DSMLevelFB,DSMModeFB] = MassageDistributeFunc(IVILevel,IVIMode,MassageLevel,MassageMode,LostFlag,ModeEEPROM) [function]
  state MassageActive
    note: 进入按摩功能
    state MassageClose
      note: 按摩关闭
      state MassageConsecutiveCount_T1 [parallel]
        settings: executionOrder=2
        note: 按摩连续开启时间计时
        (default) -> (junction 182)
        MassageConsecutiveCount_T1 -> (junction 182)
        (junction 182) -> (junction 184) [order 1] : /*是否由按摩开启状态进入*/
            | [MassageOpenFlag == TRUE]
        (junction 184) -> (junction 188) [order 1] : /*T1计时是否已到阈值*/
            | [T1timer < T1Max]
        (junction 182) -> (junction 193) [order 2]
        (junction 184) -> (junction 323) [order 2] : {T1timer = T1Max;}
        (junction 188) -> (junction 190) : {T1timer ++;}
        (junction 323) -> (junction 324) [order 1] : /*T2没有启动计时，避免T1计时到阈值后T2停止计时mantis：7343*/
            | [0 == T2timer]
        (junction 323) -> (junction 186) [order 2]
        (junction 324) -> (junction 327) : {T3timer = 0;
            | T4timer = 0;
            | AcTCount = 0;}
        (junction 186) -> (junction 193)
        (junction 327) -> (junction 186)
        (junction 190) -> (junction 327)
        (junction 193) -> (junction 196)
      state MassageStopCount_T2 [parallel]
        settings: executionOrder=1
        note: 按摩不响应时间计时
        (default) -> (junction 200)
        MassageStopCount_T2 -> (junction 200)
        (junction 200) -> (junction 202) [order 1] : /*超时关闭次数是否到阈值*/
            | [AcTCount < D_ActMax]
        (junction 202) -> (junction 205) [order 1] : /*T4计时是否到阈值*/
            | [T4timer < T4Max]
        (junction 205) -> (junction 207) [order 1] : [AutoOffFlag == FALSE]
        (junction 200) -> (junction 230) [order 2]
        (junction 202) -> (junction 232) [order 2]
        (junction 205) -> (junction 300) [order 2]
        (junction 207) -> (junction 302)
        (junction 232) -> (junction 230)
        (junction 230) -> (junction 238)
        (junction 238) -> (junction 240) [order 1] : /*T2计时是否到阈值*/
            | [T2timer < T2Max]
        (junction 300) -> (junction 305) [order 1] : [Timer_TutoOff >= 20]
        (junction 305) -> (junction 302) [order 1] : [hasChangedTo(Mas_IVI_MassageLevel_Req, enMassageLevel_IVI.EN_L1) ...
            | || hasChangedTo(Mas_IVI_MassageLevel_Req, enMassageLevel_IVI.EN_L2) ...
            | || hasChangedTo(Mas_IVI_MassageLevel_Req, enMassageLevel_IVI.EN_L3)]
        (junction 238) -> (junction 245) [order 2] : /*A1，T2保持，其余清除；报文正常转发*/
            | {AutoOffFlag = FALSE;
            | T2timer = 0;
            | T3timer = 0;
            | T4timer = 0;
            | AcTCount = 0;
            | [MassageLevel_Req, ...
            | MassageMode_Req, ...
            | DSM_MassageLevel_FB, ...
            | DSM_MassageMode_FB]= ...
            | MassageDistributeFunc ...
            | (Mas_IVI_MassageLevel_Req, ...
            | Mas_IVI_MassageMode_Req, ...
            | Mas_Massage_LevelSts_FB, ...
            | Mas_Massage_ModeSts_FB, ...
            | Mas_Massage_0x1B_LostFlag, ...
            | Mas_SeatMassageMode)}
        (junction 240) -> (junction 242) : {T2timer ++;
            | MassageLevel_Req =  ...
            | enMassageLevel_DSM.EN_AUTO_OFF;
            | DSM_MassageLevel_FB = ...
            | enMassageLevel_DSM.EN_AUTO_OFF; }
        (junction 300) -> (junction 235) [order 2] : {Timer_TutoOff ++ ;
            | /*A2档位AutoOFF，模式保持*/
            | MassageLevel_Req =  ...
            | enMassageLevel_DSM.EN_AUTO_OFF;
            | DSM_MassageLevel_FB = ...
            | enMassageLevel_DSM.EN_AUTO_OFF; }
        (junction 305) -> (junction 315) [order 2]
        (junction 302) -> (junction 209) : {T2timer = 0;
            | /*A3正常转发*/
            | [MassageLevel_Req, ...
            | MassageMode_Req, ...
            | DSM_MassageLevel_FB, ...
            | DSM_MassageMode_FB]= ...
            | MassageDistributeFunc ...
            | (Mas_IVI_MassageLevel_Req, ...
            | Mas_IVI_MassageMode_Req, ...
            | Mas_Massage_LevelSts_FB, ...
            | Mas_Massage_ModeSts_FB, ...
            | Mas_Massage_0x1B_LostFlag, ...
            | Mas_SeatMassageMode)}
        (junction 315) -> (junction 317) [order 1] : /* 自动关闭后模式转发的处理 -与正常转发逻辑保持一致*/
            | [Mas_Massage_ModeSts_FB <= ...
            | enMassageMode_DSM.EN_MError ...
            | && Mas_Massage_LevelSts_FB != ...
            | enMassageLevel_DSM.EN_AUTO_OFF ...
            | && Mas_Massage_LevelSts_FB != ...
            | enMassageLevel_DSM.EN_OFF ...
            | && Mas_Massage_0x1B_LostFlag != TRUE]
        (junction 315) -> (junction 309) [order 2] : {DSM_MassageMode_FB = ...
            | Mas_SeatMassageMode;}
        (junction 317) -> (junction 320) : {DSM_MassageMode_FB = ...
            | Mas_Massage_ModeSts_FB;}
        (junction 242) -> (junction 245)
        (junction 235) -> (junction 242)
        (junction 309) -> (junction 235)
        (junction 320) -> (junction 309)
        (junction 209) -> (junction 320)
        (junction 245) -> (junction 249)
    state MassageOpen
      en,du:
      T3timer ++;
      T4timer ++;
      /*A3正常转发*/
      [MassageLevel_Req, ...
      MassageMode_Req, ...
      DSM_MassageLevel_FB, ...
      DSM_MassageMode_FB]= ...
      MassageDistributeFunc ...
      (Mas_IVI_MassageLevel_Req, ...
      Mas_IVI_MassageMode_Req, ...
      Mas_Massage_LevelSts_FB, ...
      Mas_Massage_ModeSts_FB, ...
      Mas_Massage_0x1B_LostFlag, ...
      Mas_SeatMassageMode)
      ex:
      MassageOpenFlag = TRUE;
      AutoOffFlag = FALSE;
      note: 按摩开启
    state MassageTimeout
      note: 按摩超时
      (default) -> (junction 258)
      MassageTimeout -> (junction 258) [order 1]
      (junction 258) -> (junction 260) [order 1] : /*是否连续开启*/
          | [T3timer >= T3Max ...
          | && T1timer < T1Max]
      (junction 258) -> (junction 264) [order 2]
      (junction 260) -> (junction 262) : {AcTCount ++;}
      (junction 262) -> (junction 264)
      (junction 264) -> (junction 267) : {ExitFlag = TRUE;}
      (junction 267) -> (junction 269)
    (default) -> MassageClose
    MassageClose -> MassageOpen : /*C1 && C4*/
        | [(hasChangedTo(Mas_Massage_LevelSts_FB, enMassageLevel_DSM.EN_L1)  ...
        | || hasChangedTo(Mas_Massage_LevelSts_FB, enMassageLevel_DSM.EN_L2) ...
        | || hasChangedTo(Mas_Massage_LevelSts_FB, enMassageLevel_DSM.EN_L3)) ...
        | && (T2timer >= T2Max || T2timer == 0)]
        | {MassageOpenFlag = FALSE;
        | T2timer = 0;
        | Timer_TutoOff = 0;}
    MassageOpen -> MassageClose [order 1] : /*C2*/
        | [Mas_Massage_LevelSts_FB == enMassageLevel_DSM.EN_OFF]
        | {T3timer = 0;
        | T1timer = 0;}
    MassageOpen -> MassageTimeout [order 2] : /*C3*/
        | [T3timer >= T3Max ...
        | || T4timer >= T4Max]
    MassageTimeout -> MassageClose [order 1] : /*C3*/
        | [ExitFlag == TRUE]
        | {ExitFlag = FALSE;
        | T3timer = 0;
        | T1timer = 0;
        | AutoOffFlag = TRUE;}
  state MassageInactive
    en:
    MassageOpenFlag = FALSE;
    ExitFlag = FALSE;
    AutoOffFlag = FALSE;
    T1timer = 0;
    T2timer = 0;
    T3timer = 0;
    T4timer = 0;
    AcTCount = 0;
    MassageLevel_Req = enMassageLevel_DSM.EN_OFF;
    DSM_MassageLevel_FB =  enMassageLevel_DSM.EN_OFF;
    MassageMode_Req = Mas_SeatMassageMode;
    du:
    /*考虑恢复出厂ModeReq*/
    MassageLevel_Req = enMassageLevel_DSM.EN_OFF;
    DSM_MassageLevel_FB =  enMassageLevel_DSM.EN_OFF;
    MassageMode_Req = Mas_SeatMassageMode;
    note: 未进入按摩功能
    note: 按摩节点无故障
    state MassageNoneFault
      en,du:
      DSM_MassageMode_FB = Mas_SeatMassageMode;
    note: 按摩节点有故障
    state MassageHaveFault
      en,du:
      DSM_MassageMode_FB = Mas_Massage_ModeSts_FB;
    (default) -> MassageNoneFault
    MassageNoneFault -> MassageHaveFault : /*Massage_ModeSts_FB
        | ==0x8:enMassageError mantis(7247)*/
        | [Mas_Massage_ModeSts_FB == enMassageMode_DSM.EN_MError]
    MassageHaveFault -> MassageNoneFault : /*Massage_ModeSts_FB
        | != 0x8:enMassageError
        | || 恢复出厂模式 == TRUE*/
        | [Mas_Massage_ModeSts_FB != enMassageMode_DSM.EN_MError ...
        | || Mas_RecoverDefaultFlag == TRUE]
  (default) -> MassageInactive
  MassageInactive -> MassageActive : /*满足CC1*/
      | [MassagePC_Flag == TRUE]
  MassageActive -> MassageHaveFault [order 1] : /*Massage_ModeSts_FB ==
      | 0x8:enMassageError*/
      | [Mas_Massage_ModeSts_FB ==enMassageMode_DSM.EN_MError]
  MassageActive -> MassageInactive [order 2] : /*不满足CC1*/
      | [MassagePC_Flag != TRUE]
  data: ButtonNum function_input double size=1; FBSts function_input double size=1; CallFB1 function_output double size=1; CallFB2 function_output double size=1; CallFB3 function_output double size=1; DSMLevelReq function_output; DSMModeReq function_output; DSMLevelFB function_output; DSMModeFB function_output; IVILevel function_input; IVIMode function_input; MassageLevel function_input; MassageMode function_input; LostFlag function_input; ModeEEPROM function_input; MassageLevel_Req output uint8; MassageMode_Req output uint8; T2timer output uint16; DSM_MassageLevel_FB output Enum: enMassageLevel_DSM; FALSE parameter; Mas_IVI_MassageLevel_Req input; Mas_IVI_MassageMode_Req input; Mas_Massage_LevelSts_FB input; Mas_RecoverDefaultFlag input; Mas_Massage_0x1B_LostFlag input; MassagePC_Flag input; T1Max input; T2Max input; T3Max input; TRUE parameter; Mas_Massage_ModeSts_FB input; T4Max input; Mas_SeatMassageMode input; DSM_MassageMode_FB output Enum: enMassageMode_DSM; T1timer output uint16; T3timer output uint32; AutoOffFlag local uint8; MassageOpenFlag local uint8; ExitFlag local uint8; T4timer output uint32; AcTCount output uint8; D_ActMax input; Timer_TutoOff local uint8

== stateflow chart Appl_MassageMode_CtrlModel/UpDataInputInfo/InputSignalProcess/MassagePreconditionDeal/MassagePreconditionDeal ==
  note: /* Note
      | 存储 模式 至EEPROM
      | 输入：1.模式 */
  state SaveMassageMode(Mode) [function]
  state TRUE
    en:
    MassagePC_Flag = TRUE;
  state Init
    en:
    MassagePC_Flag = FALSE;
  state FALSE
    en:
    MassagePC_Flag = FALSE;
    du:
    FALSE -> (junction 99) [order 1]
    (junction 99) -> (junction 104)
    (junction 104) -> (junction 106) [order 1] : [RecoverDefaultDelayTimer < 200]
    (junction 104) -> (junction 110) [order 2]
    (junction 106) -> (junction 108) : {RecoverDefaultDelayTimer ++;}
    (junction 108) -> (junction 110)
    (junction 110) -> (junction 113)
    (junction 113) -> (junction 118) [order 1] : [Mas_RecoverDefaultFlag == TRUE]
    (junction 113) -> (junction 122) [order 2]
    (junction 118) -> (junction 120) : {SaveMassageMode(enMassageMode_DSM.EN_M1)}
    (junction 120) -> (junction 122)
    (junction 122) -> (junction 125)
  Init -> TRUE [order 8] : /*电源档位 == ON
      | && (发动机运行状态 == TRUE || 整车运行状态 == TRUE)
      | && Massage_ModeSts_FB != 0x8:enMassageError
      | && 按摩配置字 == TRUE
      | && 车辆类型 == P20
      | && 恢复出厂模式 != TRUE
      | && 电压处于正常模式
      | /MassagePCStopReason = 0x0:enNone;*/
      | [Mas_PowerMode == enPowerModeSts.EN_ON ...
      | && (Mas_VehicleRunFlag == TRUE || Mas_EngineRunFlag == TRUE)  ...
      | && Mas_MassageMode_FB != enMassageMode_DSM.EN_MError ...
      | && Mas_SeatMassageCfg == TRUE ...
      | && Mas_VehiclePrm == enVehTypePrm.enP20 ...
      | && Mas_RecoverDefaultFlag != TRUE ...
      | && Mas_VoltMode == enFinalPowerMode.EN_NORMAL_VOLT]
      | {MassagePCStopReason = enMasReason.enNone}
  (default) -> Init
  FALSE -> TRUE [order 1] : /*电源档位 == ON
      | && (发动机运行状态 == TRUE || 整车运行状态 == TRUE)
      | && Massage_ModeSts_FB != 0x8:enMassageError
      | && 按摩配置字 == TRUE
      | && 车辆类型 == P20
      | && 恢复出厂模式 != TRUE
      | && 电压处于正常模式
      | /MassagePCStopReason = 0x0:enNone;*/
      | [Mas_PowerMode == enPowerModeSts.EN_ON ...
      | && (Mas_VehicleRunFlag == TRUE || Mas_EngineRunFlag == TRUE)  ...
      | && Mas_MassageMode_FB != enMassageMode_DSM.EN_MError ...
      | && Mas_SeatMassageCfg == TRUE ...
      | && Mas_VehiclePrm == enVehTypePrm.enP20 ...
      | && (Mas_RecoverDefaultFlag != TRUE && RecoverDefaultDelayTimer >= 200) ...
      | && Mas_VoltMode == enFinalPowerMode.EN_NORMAL_VOLT]
      | {MassagePCStopReason = enMasReason.enNone}
  Init -> FALSE [order 1] : /*MassagePC未置位原因 Mas_PowerMode 不满足条件*/
      | [Mas_PowerMode != enPowerModeSts.EN_ON]
      | {MassagePCStopReason = enMasReason.enPowerError}
  TRUE -> FALSE [order 1] : /*MassagePC未置位原因 Mas_PowerMode 不满足条件*/
      | [Mas_PowerMode != enPowerModeSts.EN_ON]
      | {MassagePCStopReason = enMasReason.enPowerError}
  TRUE -> FALSE [order 2] : /*MassagePC未置位原因 Mas_VehicleRunFlag 不满足条件*/
      | [Mas_VehicleRunFlag != TRUE && Mas_EngineRunFlag != TRUE]
      | {MassagePCStopReason = enMasReason.enRunError}
  Init -> FALSE [order 2] : /*MassagePC未置位原因 Mas_VehicleRunFlag 不满足条件*/
      | [Mas_VehicleRunFlag != TRUE && Mas_EngineRunFlag != TRUE]
      | {MassagePCStopReason = enMasReason.enRunError}
  TRUE -> FALSE [order 3] : /*MassagePC未置位原因 ：Mas_MassageMode_FB 不满足条件*/
      | [Mas_MassageMode_FB == enMassageMode_DSM.EN_MError]
      | {MassagePCStopReason = enMasReason.enNodeError}
  Init -> FALSE [order 3] : /*MassagePC未置位原因 ：Mas_MassageMode_FB 不满足条件*/
      | [Mas_MassageMode_FB == enMassageMode_DSM.EN_MError]
      | {MassagePCStopReason = enMasReason.enNodeError}
  TRUE -> FALSE [order 4] : /*MassagePC未置位原因 ：Mas_SeatMassageCfg不满足条件*/
      | [Mas_SeatMassageCfg != TRUE]
      | {MassagePCStopReason = enMasReason.enConfigError}
  Init -> FALSE [order 4] : /*MassagePC未置位原因 ：Mas_SeatMassageCfg不满足条件*/
      | [Mas_SeatMassageCfg != TRUE]
      | {MassagePCStopReason = enMasReason.enConfigError}
  TRUE -> FALSE [order 5] : /*MassagePC未置位原因 ：Mas_VehiclePrm 不满足条件*/
      | [Mas_VehiclePrm != enVehTypePrm.enP20]
      | {MassagePCStopReason = enMasReason.enCarTypeError}
  Init -> FALSE [order 5] : /*MassagePC未置位原因 ：Mas_VehiclePrm 不满足条件*/
      | [Mas_VehiclePrm != enVehTypePrm.enP20]
      | {MassagePCStopReason = enMasReason.enCarTypeError}
  Init -> FALSE [order 6] : /*MassagePC未置位原因 ：Mas_RecoverDefaultFlag 不满足条件  */
      | [Mas_RecoverDefaultFlag == TRUE]
      | {MassagePCStopReason = enMasReason.enRecoverError}
  TRUE -> FALSE [order 6] : /*MassagePC未置位原因 ：Mas_RecoverDefaultFlag 不满足条件  */
      | [Mas_RecoverDefaultFlag == TRUE]
      | {MassagePCStopReason = enMasReason.enRecoverError;
      | RecoverDefaultDelayTimer = 0;
      | SaveMassageMode(enMassageMode_DSM.EN_M1)}
  Init -> FALSE [order 7] : /*MassagePC未置位原因 ：Mas_VoltMode 不满足条件*/
      | [Mas_VoltMode != enFinalPowerMode.EN_NORMAL_VOLT]
      | {MassagePCStopReason = enMasReason.enPowerModeError}
  TRUE -> FALSE [order 7] : /*MassagePC未置位原因 ：Mas_VoltMode 不满足条件*/
      | [Mas_VoltMode != enFinalPowerMode.EN_NORMAL_VOLT]
      | {MassagePCStopReason = enMasReason.enPowerModeError}
  data: Mode function_input; TRUE parameter; FALSE parameter; Mas_PowerMode input; Mas_RecoverDefaultFlag input; Mas_VehiclePrm input; Mas_VehicleRunFlag input; Mas_SeatMassageCfg input; Mas_MassageMode_FB input; Mas_VoltMode input; Mas_EngineRunFlag input; MassagePC_Flag output uint8; MassagePCStopReason output uint8; RecoverDefaultDelayTimer local uint16

== stateflow chart Appl_MassageMode_CtrlModel/UpDataInputInfo/InputSignalProcess/ThresholdDeal/ThresholdDeal/MemCallWaitFBFunc/Chart ==
  (default) -> (junction 3)
  (junction 3) -> (junction 5) : {CallFB1 = enMemCallFb.EN_MemCallFb_NULL;
      | CallFB2 = enMemCallFb.EN_MemCallFb_NULL;
      | CallFB3 = enMemCallFb.EN_MemCallFb_NULL;}
  (junction 5) -> (junction 7) [order 1] : /* 调用位置1进行中 */
      | [ButtonNum == 1]
  (junction 5) -> (junction 14) [order 2]
  (junction 7) -> (junction 9) : {CallFB1 = FBSts;}
  (junction 14) -> (junction 16) [order 1] : /* 调用位置2 进行中 */
      | [ButtonNum == 2]
  (junction 14) -> (junction 20) [order 2] : {CallFB3 = FBSts;}
  (junction 16) -> (junction 18) : {CallFB2 = FBSts;}
  (junction 18) -> (junction 20)
  (junction 9) -> (junction 18)
  (junction 20) -> (junction 27)
  data: ButtonNum input uint8; FBSts input Enum: enMemCallFb; CallFB1 output Enum: enMemCallFb; CallFB2 output Enum: enMemCallFb; CallFB3 output Enum: enMemCallFb
